simulink model "lab9"  (Simulink 7.9)
settings: Solver=ode45  StartTime=0.0  StopTime=10.0  RelTol=1e-3
settings Model: Creator=Mihail  LastModifiedBy=Mihail

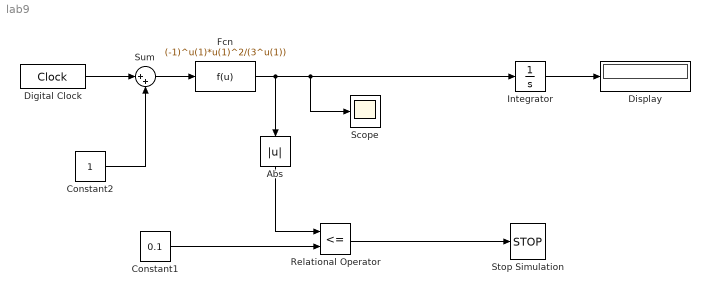
== system lab9 ==
  Abs : Abs
  Constant1 : Constant  Value=0.1
  Constant2 : Constant
  Digital Clock : DigitalClock
  Display : Display
  Fcn : Fcn  Expr=(-1)^u(1)*u(1)^2/(3^u(1))
  Integrator : Integrator
  Relational Operator : RelationalOperator  Operator=<=  OutDataTypeStr=boolean
  Scope : Scope
  Stop Simulation : Stop
  Sum : Sum  Inputs=|++
  wires:
  Integrator/1 -> Display/1
  Fcn/1 -> Abs/1, Integrator/1, Scope/1
  Constant1/1 -> Relational Operator/2
  Abs/1 -> Relational Operator/1
  Relational Operator/1 -> Stop Simulation/1
  Digital Clock/1 -> Sum/1
  Constant2/1 -> Sum/2
  Sum/1 -> Fcn/1
